simulink model "scheme_batch_op_regulation"  (R2025a)
settings: Solver=ode3  StartTime=0.0  StopTime=40  FixedStep=dt  RelTol=1e-3
values from neighbouring files (symbols this model uses):
  dt = 0.0001    [Planning_w_Adaptive.m]    (also in runBatchTests.m = 0.0005; tune_mrac_params.m = 0.01)
  map_scale = 0.5    [Planning_w_Adaptive.m]    (also in tune_mrac_params.m)
  N = -1 / (C_output_phi * inv(Am) * B)    [Planning_w_Adaptive.m]    (also in tune_mrac_params.m)
  op_space_pose_trajectory = zeros(4, 4, num_points)    [runBatchTests.m]
  waypoints = pathObj.States(:, 1:2)    [Planning_w_Adaptive.m]    (also in tune_mrac_params.m)
  x0 = zeros(10, 1)    [LQR_Control_generated.m]    (also in PID_LQR_PI_Loop.m = zeros(14, 1); Planning_w_Adaptive.m)
undefined symbols (not defined in the file or in its folder): control_params, initial_positions_rad, manipulator_time_vector, p, X, Y, Z
libraries: sm_lib x179, nesl_utility x28, fl_lib x3
(part 4 of 5)

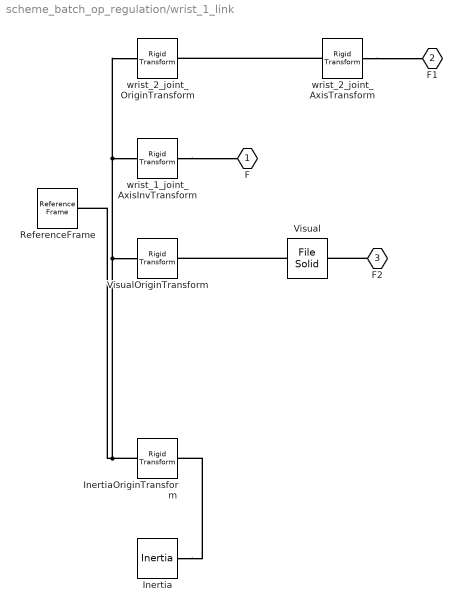
== system scheme_batch_op_regulation/wrist_1_link ==
  Inertia : sm_lib/Body Elements/Inertia  InertiaType=Custom  Mass=1.37  MassUnits=kg  CenterOfMass=[0, 0, 0]  CenterOfMassUnits=m  MomentsOfInertia=[0.00165491, 0.00126279, 0.00135962]  MomentsOfInertiaUnits=kg*m^2  ProductsOfInertia=[-0.00010157, -2.819999999999998e-06, 4.380000000000001e-06]  ProductsOfInertiaUnits=kg*m^2  GraphicType=None  MarkerShape=Inertia  MarkerSize=20  GraphicVisPropType=SimpleVisualProperties  GraphicDiffuseColor=[0.5 0.5 0.5]  GraphicOpacity=1  GraphicSpecularColor=[0.5 0.5 0.5 1.0]  GraphicAmbientColor=[0.15 0.15 0.15 1.0]  GraphicEmissiveColor=[0.0 0.0 0.0 1.0]  GraphicShininess=75
  InertiaOriginTransform : sm_lib/Frames and Transforms/Rigid Transform  RotationMethod=RotationSequence  FollAlignAxisA=+X  BaseAlignAxisA=+Y  FollAlignAxisB=+Y  BaseAlignAxisB=+Z  RotationStandardAxis=+Z  RotationAngle=0  RotationAngleUnits=deg  RotationArbitraryAxis=[0 0 1]  RotationSequenceAxes=BaseAxes  RotationSequence=XYZ  RotationSequenceAngles=[0, 0, 0]  RotationSequenceAnglesUnits=rad  RotationMatrix=[1 0 0;0 1 0;0 0 1]  Quaternion=[1 0 0 0]  TranslationMethod=Cartesian  TranslationCartesianOffset=[0, -0.01634, -0.0018]  TranslationCartesianOffsetUnits=m  TranslationStandardAxis=+Z  TranslationStandardOffset=0  TranslationStandardOffsetUnits=m  TranslationROffset=0  TranslationROffsetUnits=m  TranslationThetaOffset=0  TranslationThetaOffsetUnits=deg  TranslationZOffset=0  TranslationZOffsetUnits=m
  ReferenceFrame : sm_lib/Frames and Transforms/Reference Frame
  Visual : sm_lib/Body Elements/File Solid  ExtGeomFileName=C:\Users\robyr\Desktop\MatDrive\Published\FieldProject\generated\ros_packages\ur_description\meshes\ur5e\visual\wrist1.dae  UnitType=Custom  ExtGeomFileUnits=m  StepReaderType=HEX  ExportConvexHullGeometry=on  InertiaType=Custom  BasedOnType=DensityFromFile  Density=1000  DensityUnits=kg/m^3  Mass=0  MassUnits=kg  CenterOfMass=[0, 0, 0]  CenterOfMassUnits=m  MomentsOfInertia=[0, 0, 0]  MomentsOfInertiaUnits=kg*m^2  ProductsOfInertia=[0, 0, 0]  ProductsOfInertiaUnits=kg*m^2  GraphicType=FromGeometry  MarkerShape=Sphere  MarkerSize=10  GraphicVisPropType=SimpleVisualProperties  GraphicDiffuseColor=[0.5, 0.5, 0.5]  GraphicOpacity=1  GraphicSpecularColor=[0.5 0.5 0.5 1.0]  GraphicAmbientColor=[0.15 0.15 0.15 1.0]  GraphicEmissiveColor=[0.0 0.0 0.0 1.0]  GraphicShininess=75  DoExposeReferenceFrame=on  SerializedFrames=<Frames/>
  VisualOriginTransform : sm_lib/Frames and Transforms/Rigid Transform  RotationMethod=RotationSequence  FollAlignAxisA=+X  BaseAlignAxisA=+Y  FollAlignAxisB=+Y  BaseAlignAxisB=+Z  RotationStandardAxis=+Z  RotationAngle=0  RotationAngleUnits=deg  RotationArbitraryAxis=[0 0 1]  RotationSequenceAxes=BaseAxes  RotationSequence=XYZ  RotationSequenceAngles=[1.570796326794897, 0, 0]  RotationSequenceAnglesUnits=rad  RotationMatrix=[1 0 0;0 1 0;0 0 1]  Quaternion=[1 0 0 0]  TranslationMethod=Cartesian  TranslationCartesianOffset=[0, 0, -0.127]  TranslationCartesianOffsetUnits=m  TranslationStandardAxis=+Z  TranslationStandardOffset=0  TranslationStandardOffsetUnits=m  TranslationROffset=0  TranslationROffsetUnits=m  TranslationThetaOffset=0  TranslationThetaOffsetUnits=deg  TranslationZOffset=0  TranslationZOffsetUnits=m
  wrist_1_joint_AxisInvTransform : sm_lib/Frames and Transforms/Rigid Transform  RotationMethod=ArbitraryAxis  FollAlignAxisA=+X  BaseAlignAxisA=+Y  FollAlignAxisB=+Y  BaseAlignAxisB=+Z  RotationStandardAxis=+Z  RotationAngle=0  RotationAngleUnits=rad  RotationArbitraryAxis=[1, 0, 0]  RotationSequenceAxes=FollowerAxes  RotationSequence=XYX  RotationSequenceAngles=[0 0 0]  RotationSequenceAnglesUnits=deg  RotationMatrix=[1 0 0;0 1 0;0 0 1]  Quaternion=[1 0 0 0]  TranslationMethod=Cartesian  TranslationCartesianOffset=[0, 0, 0]  TranslationCartesianOffsetUnits=m  TranslationStandardAxis=+Z  TranslationStandardOffset=0  TranslationStandardOffsetUnits=m  TranslationROffset=0  TranslationROffsetUnits=m  TranslationThetaOffset=0  TranslationThetaOffsetUnits=deg  TranslationZOffset=0  TranslationZOffsetUnits=m
  wrist_2_joint_AxisTransform : sm_lib/Frames and Transforms/Rigid Transform  RotationMethod=ArbitraryAxis  FollAlignAxisA=+X  BaseAlignAxisA=+Y  FollAlignAxisB=+Y  BaseAlignAxisB=+Z  RotationStandardAxis=+Z  RotationAngle=0  RotationAngleUnits=rad  RotationArbitraryAxis=[1, 0, 0]  RotationSequenceAxes=FollowerAxes  RotationSequence=XYX  RotationSequenceAngles=[0 0 0]  RotationSequenceAnglesUnits=deg  RotationMatrix=[1 0 0;0 1 0;0 0 1]  Quaternion=[1 0 0 0]  TranslationMethod=Cartesian  TranslationCartesianOffset=[0, 0, 0]  TranslationCartesianOffsetUnits=m  TranslationStandardAxis=+Z  TranslationStandardOffset=0  TranslationStandardOffsetUnits=m  TranslationROffset=0  TranslationROffsetUnits=m  TranslationThetaOffset=0  TranslationThetaOffsetUnits=deg  TranslationZOffset=0  TranslationZOffsetUnits=m
  wrist_2_joint_OriginTransform : sm_lib/Frames and Transforms/Rigid Transform  RotationMethod=RotationSequence  FollAlignAxisA=+X  BaseAlignAxisA=+Y  FollAlignAxisB=+Y  BaseAlignAxisB=+Z  RotationStandardAxis=+Z  RotationAngle=0  RotationAngleUnits=deg  RotationArbitraryAxis=[0 0 1]  RotationSequenceAxes=BaseAxes  RotationSequence=XYZ  RotationSequenceAngles=[1.570796327, -0, 0]  RotationSequenceAnglesUnits=rad  RotationMatrix=[1 0 0;0 1 0;0 0 1]  Quaternion=[1 0 0 0]  TranslationMethod=Cartesian  TranslationCartesianOffset=[0, -0.0997, -2.044881182297852e-11]  TranslationCartesianOffsetUnits=m  TranslationStandardAxis=+Z  TranslationStandardOffset=0  TranslationStandardOffsetUnits=m  TranslationROffset=0  TranslationROffsetUnits=m  TranslationThetaOffset=0  TranslationThetaOffsetUnits=deg  TranslationZOffset=0  TranslationZOffsetUnits=m
  F : PMIOPort  Side=Left
  F1 : PMIOPort  Port=2  Side=Right
  F2 : PMIOPort  Port=3  Side=Left
  connections:
  Inertia/RConn1 -- InertiaOriginTransform/RConn1
  ReferenceFrame/RConn1 -- InertiaOriginTransform/LConn1 -- wrist_1_joint_AxisInvTransform/LConn1 -- wrist_2_joint_OriginTransform/LConn1 -- VisualOriginTransform/LConn1
  Visual/RConn1 -- VisualOriginTransform/RConn1
  wrist_1_joint_AxisInvTransform/RConn1 -- F/RConn1
  wrist_2_joint_AxisTransform/RConn1 -- F1/RConn1
  wrist_2_joint_AxisTransform/LConn1 -- wrist_2_joint_OriginTransform/RConn1
  F2/RConn1 -- Visual/LConn1

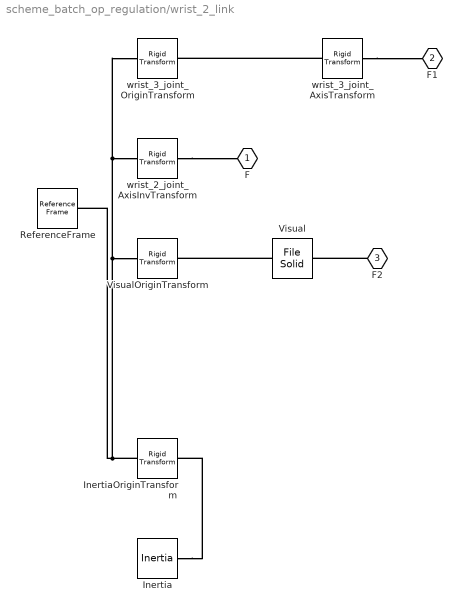
== system scheme_batch_op_regulation/wrist_2_link ==
  Inertia : sm_lib/Body Elements/Inertia  InertiaType=Custom  Mass=1.3  MassUnits=kg  CenterOfMass=[0, 0, 0]  CenterOfMassUnits=m  MomentsOfInertia=[0.00135617, 0.00096614, 0.00127827]  MomentsOfInertiaUnits=kg*m^2  ProductsOfInertia=[5.048000000000011e-05, 2.739999999999998e-06, 4.440000000000001e-06]  ProductsOfInertiaUnits=kg*m^2  GraphicType=None  MarkerShape=Inertia  MarkerSize=20  GraphicVisPropType=SimpleVisualProperties  GraphicDiffuseColor=[0.5 0.5 0.5]  GraphicOpacity=1  GraphicSpecularColor=[0.5 0.5 0.5 1.0]  GraphicAmbientColor=[0.15 0.15 0.15 1.0]  GraphicEmissiveColor=[0.0 0.0 0.0 1.0]  GraphicShininess=75
  InertiaOriginTransform : sm_lib/Frames and Transforms/Rigid Transform  RotationMethod=RotationSequence  FollAlignAxisA=+X  BaseAlignAxisA=+Y  FollAlignAxisB=+Y  BaseAlignAxisB=+Z  RotationStandardAxis=+Z  RotationAngle=0  RotationAngleUnits=deg  RotationArbitraryAxis=[0 0 1]  RotationSequenceAxes=BaseAxes  RotationSequence=XYZ  RotationSequenceAngles=[0, 0, 0]  RotationSequenceAnglesUnits=rad  RotationMatrix=[1 0 0;0 1 0;0 0 1]  Quaternion=[1 0 0 0]  TranslationMethod=Cartesian  TranslationCartesianOffset=[0, 0.01634, -0.0018]  TranslationCartesianOffsetUnits=m  TranslationStandardAxis=+Z  TranslationStandardOffset=0  TranslationStandardOffsetUnits=m  TranslationROffset=0  TranslationROffsetUnits=m  TranslationThetaOffset=0  TranslationThetaOffsetUnits=deg  TranslationZOffset=0  TranslationZOffsetUnits=m
  ReferenceFrame : sm_lib/Frames and Transforms/Reference Frame
  Visual : sm_lib/Body Elements/File Solid  ExtGeomFileName=C:\Users\robyr\Desktop\MatDrive\Published\FieldProject\generated\ros_packages\ur_description\meshes\ur5e\visual\wrist2.dae  UnitType=Custom  ExtGeomFileUnits=m  StepReaderType=HEX  ExportConvexHullGeometry=on  InertiaType=Custom  BasedOnType=DensityFromFile  Density=1000  DensityUnits=kg/m^3  Mass=0  MassUnits=kg  CenterOfMass=[0, 0, 0]  CenterOfMassUnits=m  MomentsOfInertia=[0, 0, 0]  MomentsOfInertiaUnits=kg*m^2  ProductsOfInertia=[0, 0, 0]  ProductsOfInertiaUnits=kg*m^2  GraphicType=FromGeometry  MarkerShape=Sphere  MarkerSize=10  GraphicVisPropType=SimpleVisualProperties  GraphicDiffuseColor=[0.5, 0.5, 0.5]  GraphicOpacity=1  GraphicSpecularColor=[0.5 0.5 0.5 1.0]  GraphicAmbientColor=[0.15 0.15 0.15 1.0]  GraphicEmissiveColor=[0.0 0.0 0.0 1.0]  GraphicShininess=75  DoExposeReferenceFrame=on  SerializedFrames=<Frames/>
  VisualOriginTransform : sm_lib/Frames and Transforms/Rigid Transform  RotationMethod=RotationSequence  FollAlignAxisA=+X  BaseAlignAxisA=+Y  FollAlignAxisB=+Y  BaseAlignAxisB=+Z  RotationStandardAxis=+Z  RotationAngle=0  RotationAngleUnits=deg  RotationArbitraryAxis=[0 0 1]  RotationSequenceAxes=BaseAxes  RotationSequence=XYZ  RotationSequenceAngles=[0, 0, 0]  RotationSequenceAnglesUnits=rad  RotationMatrix=[1 0 0;0 1 0;0 0 1]  Quaternion=[1 0 0 0]  TranslationMethod=Cartesian  TranslationCartesianOffset=[0, 0, -0.0997]  TranslationCartesianOffsetUnits=m  TranslationStandardAxis=+Z  TranslationStandardOffset=0  TranslationStandardOffsetUnits=m  TranslationROffset=0  TranslationROffsetUnits=m  TranslationThetaOffset=0  TranslationThetaOffsetUnits=deg  TranslationZOffset=0  TranslationZOffsetUnits=m
  wrist_2_joint_AxisInvTransform : sm_lib/Frames and Transforms/Rigid Transform  RotationMethod=ArbitraryAxis  FollAlignAxisA=+X  BaseAlignAxisA=+Y  FollAlignAxisB=+Y  BaseAlignAxisB=+Z  RotationStandardAxis=+Z  RotationAngle=0  RotationAngleUnits=rad  RotationArbitraryAxis=[1, 0, 0]  RotationSequenceAxes=FollowerAxes  RotationSequence=XYX  RotationSequenceAngles=[0 0 0]  RotationSequenceAnglesUnits=deg  RotationMatrix=[1 0 0;0 1 0;0 0 1]  Quaternion=[1 0 0 0]  TranslationMethod=Cartesian  TranslationCartesianOffset=[0, 0, 0]  TranslationCartesianOffsetUnits=m  TranslationStandardAxis=+Z  TranslationStandardOffset=0  TranslationStandardOffsetUnits=m  TranslationROffset=0  TranslationROffsetUnits=m  TranslationThetaOffset=0  TranslationThetaOffsetUnits=deg  TranslationZOffset=0  TranslationZOffsetUnits=m
  wrist_3_joint_AxisTransform : sm_lib/Frames and Transforms/Rigid Transform  RotationMethod=ArbitraryAxis  FollAlignAxisA=+X  BaseAlignAxisA=+Y  FollAlignAxisB=+Y  BaseAlignAxisB=+Z  RotationStandardAxis=+Z  RotationAngle=0  RotationAngleUnits=rad  RotationArbitraryAxis=[1, 0, 0]  RotationSequenceAxes=FollowerAxes  RotationSequence=XYX  RotationSequenceAngles=[0 0 0]  RotationSequenceAnglesUnits=deg  RotationMatrix=[1 0 0;0 1 0;0 0 1]  Quaternion=[1 0 0 0]  TranslationMethod=Cartesian  TranslationCartesianOffset=[0, 0, 0]  TranslationCartesianOffsetUnits=m  TranslationStandardAxis=+Z  TranslationStandardOffset=0  TranslationStandardOffsetUnits=m  TranslationROffset=0  TranslationROffsetUnits=m  TranslationThetaOffset=0  TranslationThetaOffsetUnits=deg  TranslationZOffset=0  TranslationZOffsetUnits=m
  wrist_3_joint_OriginTransform : sm_lib/Frames and Transforms/Rigid Transform  RotationMethod=RotationSequence  FollAlignAxisA=+X  BaseAlignAxisA=+Y  FollAlignAxisB=+Y  BaseAlignAxisB=+Z  RotationStandardAxis=+Z  RotationAngle=0  RotationAngleUnits=deg  RotationArbitraryAxis=[0 0 1]  RotationSequenceAxes=BaseAxes  RotationSequence=XYZ  RotationSequenceAngles=[-1.570796327, 1.224646799147353e-16, -1.224646799147353e-16]  RotationSequenceAnglesUnits=rad  RotationMatrix=[1 0 0;0 1 0;0 0 1]  Quaternion=[1 0 0 0]  TranslationMethod=Cartesian  TranslationCartesianOffset=[0, 0.09959999999999999, -2.042830148012698e-11]  TranslationCartesianOffsetUnits=m  TranslationStandardAxis=+Z  TranslationStandardOffset=0  TranslationStandardOffsetUnits=m  TranslationROffset=0  TranslationROffsetUnits=m  TranslationThetaOffset=0  TranslationThetaOffsetUnits=deg  TranslationZOffset=0  TranslationZOffsetUnits=m
  F : PMIOPort  Side=Left
  F1 : PMIOPort  Port=2  Side=Right
  F2 : PMIOPort  Port=3  Side=Left
  connections:
  Inertia/RConn1 -- InertiaOriginTransform/RConn1
  ReferenceFrame/RConn1 -- InertiaOriginTransform/LConn1 -- wrist_2_joint_AxisInvTransform/LConn1 -- wrist_3_joint_OriginTransform/LConn1 -- VisualOriginTransform/LConn1
  Visual/RConn1 -- VisualOriginTransform/RConn1
  wrist_2_joint_AxisInvTransform/RConn1 -- F/RConn1
  wrist_3_joint_AxisTransform/RConn1 -- F1/RConn1
  wrist_3_joint_AxisTransform/LConn1 -- wrist_3_joint_OriginTransform/RConn1
  F2/RConn1 -- Visual/LConn1

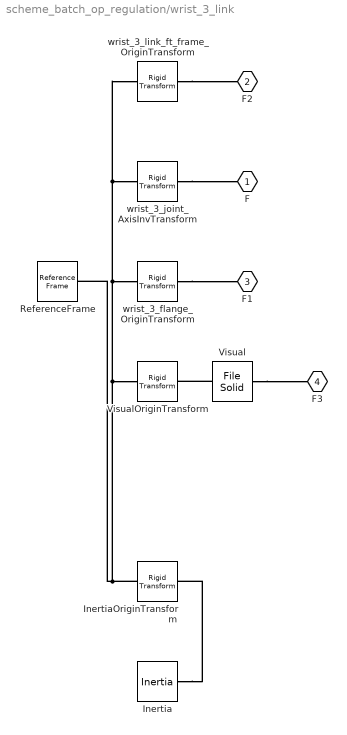
== system scheme_batch_op_regulation/wrist_3_link ==
  Inertia : sm_lib/Body Elements/Inertia  InertiaType=Custom  Mass=0.365  MassUnits=kg  CenterOfMass=[0, 0, 0]  CenterOfMassUnits=m  MomentsOfInertia=[0.00018694, 0.00018908, 0.00025756]  MomentsOfInertiaUnits=kg*m^2  ProductsOfInertia=[-9.2e-07, -1.7e-07, 5.999999999999999e-08]  ProductsOfInertiaUnits=kg*m^2  GraphicType=None  MarkerShape=Inertia  MarkerSize=20  GraphicVisPropType=SimpleVisualProperties  GraphicDiffuseColor=[0.5 0.5 0.5]  GraphicOpacity=1  GraphicSpecularColor=[0.5 0.5 0.5 1.0]  GraphicAmbientColor=[0.15 0.15 0.15 1.0]  GraphicEmissiveColor=[0.0 0.0 0.0 1.0]  GraphicShininess=75
  InertiaOriginTransform : sm_lib/Frames and Transforms/Rigid Transform  RotationMethod=RotationSequence  FollAlignAxisA=+X  BaseAlignAxisA=+Y  FollAlignAxisB=+Y  BaseAlignAxisB=+Z  RotationStandardAxis=+Z  RotationAngle=0  RotationAngleUnits=deg  RotationArbitraryAxis=[0 0 1]  RotationSequenceAxes=BaseAxes  RotationSequence=XYZ  RotationSequenceAngles=[0, 0, 0]  RotationSequenceAnglesUnits=rad  RotationMatrix=[1 0 0;0 1 0;0 0 1]  Quaternion=[1 0 0 0]  TranslationMethod=Cartesian  TranslationCartesianOffset=[0, 0, -0.001159]  TranslationCartesianOffsetUnits=m  TranslationStandardAxis=+Z  TranslationStandardOffset=0  TranslationStandardOffsetUnits=m  TranslationROffset=0  TranslationROffsetUnits=m  TranslationThetaOffset=0  TranslationThetaOffsetUnits=deg  TranslationZOffset=0  TranslationZOffsetUnits=m
  ReferenceFrame : sm_lib/Frames and Transforms/Reference Frame
  Visual : sm_lib/Body Elements/File Solid  ExtGeomFileName=C:\Users\robyr\Desktop\MatDrive\Published\FieldProject\generated\ros_packages\ur_description\meshes\ur5e\visual\wrist3.dae  UnitType=Custom  ExtGeomFileUnits=m  StepReaderType=HEX  ExportConvexHullGeometry=on  InertiaType=Custom  BasedOnType=DensityFromFile  Density=1000  DensityUnits=kg/m^3  Mass=0  MassUnits=kg  CenterOfMass=[0, 0, 0]  CenterOfMassUnits=m  MomentsOfInertia=[0, 0, 0]  MomentsOfInertiaUnits=kg*m^2  ProductsOfInertia=[0, 0, 0]  ProductsOfInertiaUnits=kg*m^2  GraphicType=FromGeometry  MarkerShape=Sphere  MarkerSize=10  GraphicVisPropType=SimpleVisualProperties  GraphicDiffuseColor=[0.5, 0.5, 0.5]  GraphicOpacity=1  GraphicSpecularColor=[0.5 0.5 0.5 1.0]  GraphicAmbientColor=[0.15 0.15 0.15 1.0]  GraphicEmissiveColor=[0.0 0.0 0.0 1.0]  GraphicShininess=75  DoExposeReferenceFrame=on  SerializedFrames=<Frames/>
  VisualOriginTransform : sm_lib/Frames and Transforms/Rigid Transform  RotationMethod=RotationSequence  FollAlignAxisA=+X  BaseAlignAxisA=+Y  FollAlignAxisB=+Y  BaseAlignAxisB=+Z  RotationStandardAxis=+Z  RotationAngle=0  RotationAngleUnits=deg  RotationArbitraryAxis=[0 0 1]  RotationSequenceAxes=BaseAxes  RotationSequence=XYZ  RotationSequenceAngles=[1.570796326794897, 0, 0]  RotationSequenceAnglesUnits=rad  RotationMatrix=[1 0 0;0 1 0;0 0 1]  Quaternion=[1 0 0 0]  TranslationMethod=Cartesian  TranslationCartesianOffset=[0, 0, -0.0989]  TranslationCartesianOffsetUnits=m  TranslationStandardAxis=+Z  TranslationStandardOffset=0  TranslationStandardOffsetUnits=m  TranslationROffset=0  TranslationROffsetUnits=m  TranslationThetaOffset=0  TranslationThetaOffsetUnits=deg  TranslationZOffset=0  TranslationZOffsetUnits=m
  wrist_3_flange_OriginTransform : sm_lib/Frames and Transforms/Rigid Transform  RotationMethod=RotationSequence  FollAlignAxisA=+X  BaseAlignAxisA=+Y  FollAlignAxisB=+Y  BaseAlignAxisB=+Z  RotationStandardAxis=+Z  RotationAngle=0  RotationAngleUnits=deg  RotationArbitraryAxis=[0 0 1]  RotationSequenceAxes=BaseAxes  RotationSequence=XYZ  RotationSequenceAngles=[-1.570796326794897, -1.570796326794897, 0]  RotationSequenceAnglesUnits=rad  RotationMatrix=[1 0 0;0 1 0;0 0 1]  Quaternion=[1 0 0 0]  TranslationMethod=Cartesian  TranslationCartesianOffset=[0, 0, 0]  TranslationCartesianOffsetUnits=m  TranslationStandardAxis=+Z  TranslationStandardOffset=0  TranslationStandardOffsetUnits=m  TranslationROffset=0  TranslationROffsetUnits=m  TranslationThetaOffset=0  TranslationThetaOffsetUnits=deg  TranslationZOffset=0  TranslationZOffsetUnits=m
  wrist_3_joint_AxisInvTransform : sm_lib/Frames and Transforms/Rigid Transform  RotationMethod=ArbitraryAxis  FollAlignAxisA=+X  BaseAlignAxisA=+Y  FollAlignAxisB=+Y  BaseAlignAxisB=+Z  RotationStandardAxis=+Z  RotationAngle=0  RotationAngleUnits=rad  RotationArbitraryAxis=[1, 0, 0]  RotationSequenceAxes=FollowerAxes  RotationSequence=XYX  RotationSequenceAngles=[0 0 0]  RotationSequenceAnglesUnits=deg  RotationMatrix=[1 0 0;0 1 0;0 0 1]  Quaternion=[1 0 0 0]  TranslationMethod=Cartesian  TranslationCartesianOffset=[0, 0, 0]  TranslationCartesianOffsetUnits=m  TranslationStandardAxis=+Z  TranslationStandardOffset=0  TranslationStandardOffsetUnits=m  TranslationROffset=0  TranslationROffsetUnits=m  TranslationThetaOffset=0  TranslationThetaOffsetUnits=deg  TranslationZOffset=0  TranslationZOffsetUnits=m
  wrist_3_link_ft_frame_OriginTransform : sm_lib/Frames and Transforms/Rigid Transform  RotationMethod=RotationSequence  FollAlignAxisA=+X  BaseAlignAxisA=+Y  FollAlignAxisB=+Y  BaseAlignAxisB=+Z  RotationStandardAxis=+Z  RotationAngle=0  RotationAngleUnits=deg  RotationArbitraryAxis=[0 0 1]  RotationSequenceAxes=BaseAxes  RotationSequence=XYZ  RotationSequenceAngles=[3.141592653589793, -0, 0]  RotationSequenceAnglesUnits=rad  RotationMatrix=[1 0 0;0 1 0;0 0 1]  Quaternion=[1 0 0 0]  TranslationMethod=Cartesian  TranslationCartesianOffset=[0, 0, 0]  TranslationCartesianOffsetUnits=m  TranslationStandardAxis=+Z  TranslationStandardOffset=0  TranslationStandardOffsetUnits=m  TranslationROffset=0  TranslationROffsetUnits=m  TranslationThetaOffset=0  TranslationThetaOffsetUnits=deg  TranslationZOffset=0  TranslationZOffsetUnits=m
  F : PMIOPort  Side=Left
  F2 : PMIOPort  Port=2  Side=Right
  F1 : PMIOPort  Port=3  Side=Right
  F3 : PMIOPort  Port=4  Side=Left
  connections:
  Inertia/RConn1 -- InertiaOriginTransform/RConn1
  ReferenceFrame/RConn1 -- InertiaOriginTransform/LConn1 -- wrist_3_joint_AxisInvTransform/LConn1 -- wrist_3_link_ft_frame_OriginTransform/LConn1 -- wrist_3_flange_OriginTransform/LConn1 -- VisualOriginTransform/LConn1
  Visual/RConn1 -- VisualOriginTransform/RConn1
  wrist_3_flange_OriginTransform/RConn1 -- F1/RConn1
  wrist_3_joint_AxisInvTransform/RConn1 -- F/RConn1
  wrist_3_link_ft_frame_OriginTransform/RConn1 -- F2/RConn1
  Visual/LConn1 -- F3/RConn1

== matlab function scheme_batch_op_regulation/MATLAB Function ==
  data: q_ref_gripper output; simscape_trajectory input; q_ref_manip output; q_op_integrated input; control_params parameter
function [q_ref_gripper,q_ref_manip ] = combine_joint_references(simscape_trajectory, q_op_integrated, control_params)
%
% This function combines a base joint-space position trajectory
% with an INTEGRATED operational-space correction command.
% It also separates the gripper command.
%
% INPUTS:
%   simscape_trajectory: (1x7) vector of joint POSITIONS from Simscape.
%   q_op_integrated:     (6x1) vector of joint POSITIONS from integrating
%                        the q_dot_command.
%
% OUTPUTS:
%   q_ref_manip:   (6x1) The final 6-joint position command.
%   q_ref_gripper: (1x1) The gripper command.
%

% --- 1. Ensure q_op_integrated is a 6x1 column vector ---
% (This helps prevent dimension mismatch errors)
q_op_integrated_col = reshape(q_op_integrated, 6, 1);

% --- 2. Extract the gripper command ---
% The 4th component of the simscape trajectory
q_ref_gripper = simscape_trajectory(4);

% --- 3. Extract the 6 manipulator joint references ---
% We take components 1, 2, 3, 5, 6, 7 and form a 6x1 column vector
q_ref_base_manip = [simscape_trajectory(1);
                    simscape_trajectory(2);
                    simscape_trajectory(3);
                    simscape_trajectory(5);
                    simscape_trajectory(6);
                    simscape_trajectory(7)];

% --- 4. Sum the base reference and the integrated correction ---
% This is the final position command for the 6 manipulator joints
q_ref_manip = q_ref_base_manip + control_params.k_op*q_op_integrated_col;

end

== matlab function scheme_batch_op_regulation/Smart LookUpTable ==
  settings: updateMethod=DISCRETE
  data: T_desired output; EUL output; t_in input; op_space_pose_trajectory parameter; manipulator_time_vector parameter; P output
function [T_desired, EUL, P] = get_pose_from_trajectory(t_in, op_space_pose_trajectory, manipulator_time_vector)
% =========================================================================
% TRAJECTORY INTERPOLATOR AND POSE SPLITTER (v4.1 - Column Vector Fix)
%
% This version transposes the EUL output to be a column vector [3x1]
% to match the expectation of downstream Simulink blocks like Demux.
% =========================================================================
    % For Coder compatibility, explicitly define the output sizes.
    P = zeros(3, 1);
    % FIX 1: Initialize EUL as a 3x1 column vector.
    EUL = zeros(3, 1);
    T_desired = eye(4);
    % Use a persistent variable to show warnings only once per simulation.
    persistent has_warned;
    if isempty(has_warned)
        has_warned = false;
    end

    % --- 1. Input Sanity Checks ---
    if isnan(t_in)
        if ~has_warned
            warning('Input time t_in is NaN. Outputting a zero pose.');
            has_warned = true;
        end
        return; % Exit with P and EUL as zeros
    end
    
    if isempty(manipulator_time_vector) || isempty(op_space_pose_trajectory)
        if ~has_warned
            warning('Trajectory data is empty. Outputting a zero pose.');
            has_warned = true;
        end
        return; % Exit with P and EUL as zeros
    end

    % --- 2. Data Formatting ---
    if isrow(manipulator_time_vector)
        manipulator_time_vector = manipulator_time_vector';
    end

    % --- 3. Interpolation ---
    if isscalar(manipulator_time_vector)
        T_interpolated = op_space_pose_trajectory(:,:,1);
    else
        num_points = size(op_space_pose_trajectory, 3);
        data_reshaped = reshape(op_space_pose_trajectory, 16, num_points)';
        
        interpolated_row = interp1(manipulator_time_vector, data_reshaped, t_in, 'linear', 'extrap');
        
        if any(isnan(interpolated_row))
             if ~has_warned
                warning('Interpolation resulted in NaN. Holding first pose as fallback.');
                has_warned = true;
             end
             T_interpolated = op_space_pose_trajectory(:,:,1);
        else
             T_interpolated = reshape(interpolated_row, 4, 4);
        end
    end
    
    % --- 4. Split the Result into Position and Euler Angles ---
    P = T_interpolated(1:3, 4);
    R = T_interpolated(1:3, 1:3);
    T_desired = T_interpolated;
    
    % FIX 2: Transpose the output of rotm2eul to create a column vector.
    EUL = rotm2eul(R, 'ZYX')'; % <-- The fix is the transpose operator '

end

== matlab function scheme_batch_op_regulation/OP SPACE CONTROLLER/MATLAB Function3 ==
  data: T_desired input; x_ballbot input; q_manip_actual input; q_dot_command output; error_pos output
function [q_dot_command,error_pos] = operational_space_controller(T_desired, x_ballbot, q_manip_actual)
% =========================================================================
% OPERATIONAL SPACE CONTROLLER (v5.1 - Final Coder-Safe Wrapper)
%
% This version correctly initializes the output variable before calling the
% extrinsic function, which is required for code generation.
% =========================================================================

    % --- Coder Directives ---
    coder.extrinsic('loadAndConfigureRobot', 'compute_op_space_velocities', 'disp');

    % --- Define persistent variables ---
    persistent robotModel p;

    % --- Initialization Block (runs only ONCE) ---
    if isempty(robotModel)
        disp('Controller Wrapper: Loading robot model and parameters...');
        robotModel = loadAndConfigureRobot('UR5e.urdf');
        p.h_U = 0.50;
        p.r_S = 0.1145;
        disp('Controller Wrapper initialized.');
    end

    % --- Main Control Call ---
    
    % FIX: Initialize the output variable with a known type and size (6x1 double).
    % This tells the Coder what to expect from the extrinsic function call.
    q_dot_command = zeros(6, 1);
    error_pos     = zeros(3, 1);
    
    % Call the single extrinsic "black box" function to do all the calculations.
    %error_pos = compute_error(robotModel, p, T_desired, x_ballbot, q_manip_actual);
    [q_dot_command,error_pos] = compute_op_space_velocities(robotModel, p, T_desired, x_ballbot, q_manip_actual);


end

== matlab function scheme_batch_op_regulation/EQ generator ==
  settings: updateMethod=DISCRETE
  data: phi_dot_c input; external_wrench input; theta_EQ output; p parameter; tau_EQ output
function [theta_EQ, tau_EQ] = compute_equilibrium_fsolve_2D(phi_dot_c, external_wrench, p)
% =========================================================================
% COMPUTE_EQUILIBRIUM_FSOLVE (v8 - Refactored)
%
% This function is now a pure solver. It calculates the equilibrium tilt
% angles (theta_EQ) and torques (tau_EQ) required to achieve a given
% wheel speed command (phi_dot_c) while under the influence of an
% external wrench.
%
% INPUTS:
%   x                - Current 10x1 state vector of the system.
%   phi_dot_c        - 2x1 desired wheel speed command [phi_dot_c_y; phi_dot_c_x].
%   external_wrench  - External forces and torques.
%   p                - Struct with system parameters.
% =========================================================================

% Use persistent variables for "warm-starting" the solver.
persistent prev_solution_x prev_solution_y;
if isempty(prev_solution_x)
    prev_solution_x = [0; 0]; % [theta_x; tau_x]
    prev_solution_y = [0; 0]; % [theta_y; tau_y]
end

%% === SECTION 1: UNPACK SPEED COMMAND ===
% The velocity command is now an input to the function.
phi_dot_c_y = phi_dot_c(1);
phi_dot_c_x = phi_dot_c(2);

%% === SECTION 2: FSOLVE FOR EQUILIBRIUM (CODER-FRIENDLY) ===
options = optimoptions('fsolve', 'Display', 'off', ...
                       'Algorithm', 'levenberg-marquardt', ...
                       'FunctionTolerance', 1e-6, ...
                       'StepTolerance', 1e-6, ...
                       'MaxIterations', 25);

% --- Solve for Pitch (Y-Z) Plane ---
up_y = [external_wrench(1); external_wrench(3); external_wrench(5)]; % [Fpx; Fpz; tau_py]
[current_solution_y, ~, exitflag_y] = fsolve(@(x_solve) equilibrium_residual_Y(x_solve, up_y, phi_dot_c_y, p), prev_solution_y, options);
if exitflag_y <= 0
    current_solution_y = prev_solution_y; % Fallback to previous solution on failure
end
theta_EQy_calc = current_solution_y(1);
tau_EQy_calc = current_solution_y(2);
prev_solution_y = current_solution_y;

% --- Solve for Roll (X-Z) Plane ---
up_x = [external_wrench(2); external_wrench(3); external_wrench(4)]; % [Fpy; Fpz; tau_px]
[current_solution_x, ~, exitflag_x] = fsolve(@(x_solve) equilibrium_residual_X(x_solve, up_x, phi_dot_c_x, p), prev_solution_x, options);
if exitflag_x <= 0
    current_solution_x = prev_solution_x; % Fallback
end
theta_EQx_calc = current_solution_x(1);
tau_EQx_calc = current_solution_x(2);
prev_solution_x = current_solution_x;

%% === SECTION 3: ASSEMBLE OUTPUTS ===
theta_EQ = [theta_EQx_calc; theta_EQy_calc];
tau_EQ = [tau_EQx_calc; tau_EQy_calc];

end

% --- Nested functions for solver residuals (unchanged) ---
function r = equilibrium_residual_Y(x_solve, upy, phi_dot_c, p)
    theta_eq = x_solve(1); tau_eq = x_solve(2);
    state_vec = [0; theta_eq; 0; 0; 0; 0; 0; 0; 0; phi_dot_c];
    tau_vec = [0; tau_eq; 0];
    wrench_vec = [upy(1); 0; upy(2); 0; upy(3)];
    dx = stateDerivative3D_with_exforce(state_vec, p, tau_vec, wrench_vec);
    r = [dx(7); dx(10)];
end

function r = equilibrium_residual_X(x_solve, upx, phi_dot_c, p)
    theta_eq = x_solve(1); tau_eq = x_solve(2);
    state_vec = [theta_eq; 0; 0; 0; 0; 0; 0; 0; phi_dot_c; 0];
    tau_vec = [tau_eq; 0; 0];
    wrench_vec = [0; upx(1); upx(2); upx(3); 0];
    dx = stateDerivative3D_with_exforce(state_vec, p, tau_vec, wrench_vec);
    r = [dx(6); dx(9)];
end

function dx = stateDerivative3D_with_exforce(x, p, tau, wrench_ext)
    % MODIFICATION 1: The function now accepts a 4th argument, 'wrench_ext',
    % which is a vector containing the external forces and torques from Simulink.
    
    % Unpack state vector (10 elements)
    theta_x = x(1); dot_theta_x = x(6);
    theta_y = x(2); dot_theta_y = x(7);
    theta_z = x(3); dot_theta_z = x(8);
    % phi_x   = x(4); % Not needed for dynamics
    % phi_y   = x(5); % Not needed for dynamics
    dot_phi_x   = x(9);
    dot_phi_y   = x(10);
    
    % Unpack input torques
    tau_x = tau(1);
    tau_y = tau(2);
    tau_z = tau(3);

     % Unpack the external wrench vector from the new input ---
    % Expected order: [F_px, F_py, F_pz, tau_px, tau_py]
    F_px   = wrench_ext(1);
    F_py   = wrench_ext(2);
    F_pz   = wrench_ext(3);
    tau_px = wrench_ext(4);
    tau_py = wrench_ext(5);

    % --- Prepare arguments for auto-generated functions ---
    % Create separate parameter vectors for each plane, now including h_app
    % Note: I_Ux is for roll, I_Uy is for pitch.
    params_arg_roll = [p.m_U,  p.I_Uy, p.I_Ux, p.l_U, p.m_S, p.I_S, p.r_S, p.g, p.h_app, p.b_theta, p.b_phi];
    params_arg_pitch = [p.m_U, p.I_Uy, p.I_Ux, p.l_U, p.m_S, p.I_S, p.r_S, p.g,p.h_app, p.b_theta, p.b_phi];
    
    external_vars_x = [F_py, F_pz, tau_px]; % For Roll dynamics
    external_vars_y = [F_px, F_pz, tau_py]; % For Pitch dynamics

    % --- X-Z Plane (Roll) Dynamics ---
    states_arg_x = [theta_x, dot_theta_x, dot_phi_x];
    inputs_arg_x = [tau_x];
    ddot_theta_x = copy_autogen_ddot_theta_x(states_arg_x, inputs_arg_x, params_arg_roll, external_vars_x);
    ddot_phi_x   = copy_autogen_ddot_phi_x(states_arg_x, inputs_arg_x, params_arg_roll, external_vars_x);
    

    % --- Y-Z Plane (Pitch) Dynamics ---
    states_arg_y = [theta_y, dot_theta_y, dot_phi_y];
    inputs_arg_y = [tau_y];
    ddot_theta_y = copy_autogen_ddot_theta_y(states_arg_y, inputs_arg_y, params_arg_pitch, external_vars_y);
    ddot_phi_y   = copy_autogen_ddot_phi_y(states_arg_y, inputs_arg_y, params_arg_pitch, external_vars_y);
    
    % --- Transversal Plane Dynamics (Yaw) ---
    % external forces at the center of the top surface are assumed not to produce yaw torque.
    ddot_theta_z = (tau_z - p.fz * dot_theta_z) / p.Iz;
    
    % --- Assemble the state derivative vector dx ---
    dx = [
        dot_theta_x;    % dx(1) = d(theta_x)/dt
        dot_theta_y;    % dx(2) = d(theta_y)/dt
        dot_theta_z;    % dx(3) = d(theta_z)/dt
        dot_phi_x;      % dx(4) = d(phi_x)/dt
        dot_phi_y;      % dx(5) = d(phi_y)/dt
        ddot_theta_x;   % dx(6) = d(dot_theta_x)/dt
        ddot_theta_y;   % dx(7) = d(dot_theta_y)/dt
        ddot_theta_z;   % dx(8) = d(dot_theta_z)/dt
        ddot_phi_x;     % dx(9) = d(dot_phi_x)/dt
        ddot_phi_y;     % dx(10)= d(dot_phi_y)/dt
    ];
end

== matlab function scheme_batch_op_regulation/LQR iHACS  ==
  settings: updateMethod=DISCRETE
  data: x input; tau output; dot_phi_cmd input; p parameter; control_params parameter; dt parameter; tau_ey output; tau_r output; tau_ex output; theta_EQ input; tau_ff_new output; tau_EQ input; sim_time input
function [tau, tau_ey, tau_r, tau_ex, tau_ff_new] = calculate_motor_torques(x, dot_phi_cmd, p, control_params, dt, theta_EQ, tau_EQ, sim_time)
% =========================================================================
% Ballbot Motor Torque Calculator (Inner Loop Controller)
%
% This function takes a desired wheel speed command and calculates the
% final motor torques using a cascaded LQR and PI control structure,
% compensated with feedforward equilibrium values.
%
% INPUTS:
%   x              (10x1): State vector
%   dot_phi_cmd    (2x1):  Desired wheel speed command [dot_phi_cmd_y; dot_phi_cmd_x]
%   p              (struct): System physical parameters
%   control_params (struct): Controller gains (K, Kp_inner, Ki_inner)
%   dt             (double): Controller sample time
%   theta_EQ       (2x1): Equilibrium tilt angles [theta_EQ_x; theta_EQ_y]
%   tau_EQ         (2x1): Equilibrium feedforward torques [tau_EQ_x; tau_EQ_y]
%   sim_time       (double): Current simulation time
% =========================================================================
persistent dot_phi_ref_old;
persistent integral_speed_error_old;
if isempty(dot_phi_ref_old)
    dot_phi_ref_old = zeros(2,1);
    integral_speed_error_old = zeros(2,1);
end

% --- UNPACK PARAMETERS, STATES, and INPUTS ---
K = control_params.K;
Kp_inner = control_params.Kp_inner;
Ki_inner = control_params.Ki_inner;
theta_x = x(1); dot_theta_x = x(6);
theta_y = x(2); dot_theta_y = x(7);
phi_x   = x(4); dot_phi_x   = x(9);
phi_y   = x(5); dot_phi_y   = x(10);
theta_EQ_x = theta_EQ(1);
theta_EQ_y = theta_EQ(2);
tau_EQ_x_raw   = tau_EQ(1);
tau_EQ_y_raw   = tau_EQ(2);

% Unpack the input speed command
dot_phi_cmd_y = dot_phi_cmd(1);
dot_phi_cmd_x = dot_phi_cmd(2);

%% --- FEEDBACK CONTROLLER (LQR + PI) ---
% --- LQR for stabilization ---
state_y = [theta_y; phi_y; dot_theta_y; dot_phi_y];
command_state_y = [theta_EQ_y; phi_y; 0; dot_phi_cmd_y];
tau_ry = -K * (state_y - command_state_y);

state_x = [theta_x; phi_x; dot_theta_x; dot_phi_x];
command_state_x = [theta_EQ_x; phi_x; 0; dot_phi_cmd_x];
tau_rx = -K * (state_x - command_state_x);
tau_z = 0;

% --- Inner PI loop speed controller ---
tau_r = [tau_rx; tau_ry; tau_z];
dx_ref = stateDerivative3D_with_exforce(x(1:10), p, tau_r, zeros(5,1));
ddot_phi_x_ref = dx_ref(9);
ddot_phi_y_ref = dx_ref(10);
dot_phi_x_ref = dot_phi_ref_old(1) + ddot_phi_x_ref * dt;
dot_phi_y_ref = dot_phi_ref_old(2) + ddot_phi_y_ref * dt;
speed_error_x = dot_phi_x_ref - dot_phi_x;
speed_error_y = dot_phi_y_ref - dot_phi_y;
int_err_vx = integral_speed_error_old(1);
int_err_vy = integral_speed_error_old(2);
tau_ex = Kp_inner * speed_error_x + Ki_inner * int_err_vx;
tau_ey = Kp_inner * speed_error_y + Ki_inner * int_err_vy;

%% --- FINAL TORQUE COMMAND ---
% Combine Feedback (LQR + PI) and Feedforward (Equilibrium Torque)
if sim_time < 0.1
    tau_EQ_x = 0;
    tau_EQ_y = 0;
else
    tau_EQ_x = tau_EQ_x_raw;
    tau_EQ_y = tau_EQ_y_raw;
end
tau_ff_new = [tau_EQ_x; tau_EQ_y; 0];
tau_x = tau_rx + tau_ex + tau_EQ_x;
tau_y = tau_ry + tau_ey + tau_EQ_y;
tau_z = 0;
tau = [tau_x; tau_y; tau_z];

% --- UPDATE PERSISTENT VARIABLES ---
integral_speed_error_old = integral_speed_error_old + [speed_error_x; speed_error_y] * dt;
dot_phi_ref_old = [dot_phi_x_ref; dot_phi_y_ref];

end

function dx = stateDerivative3D_with_exforce(x, p, tau, wrench_ext)
    % MODIFICATION 1: The function now accepts a 4th argument, 'wrench_ext',
    % which is a vector containing the external forces and torques from Simulink.
    
    % Unpack state vector (10 elements)
    theta_x = x(1); dot_theta_x = x(6);
    theta_y = x(2); dot_theta_y = x(7);
    theta_z = x(3); dot_theta_z = x(8);
    % phi_x   = x(4); % Not needed for dynamics
    % phi_y   = x(5); % Not needed for dynamics
    dot_phi_x   = x(9);
    dot_phi_y   = x(10);
    
    % Unpack input torques
    tau_x = tau(1);
    tau_y = tau(2);
    tau_z = tau(3);

     % Unpack the external wrench vector from the new input ---
    % Expected order: [F_px, F_py, F_pz, tau_px, tau_py]
    F_px   = wrench_ext(1);
    F_py   = wrench_ext(2);
    F_pz   = wrench_ext(3);
    tau_px = wrench_ext(4);
    tau_py = wrench_ext(5);

    % --- Prepare arguments for auto-generated functions ---
    % Create separate parameter vectors for each plane, now including h_app
    % Note: I_Ux is for roll, I_Uy is for pitch.
    params_arg_roll = [p.m_U,  p.I_Uy, p.I_Ux, p.l_U, p.m_S, p.I_S, p.r_S, p.g, p.h_app, p.b_theta, p.b_phi];
    params_arg_pitch = [p.m_U, p.I_Uy, p.I_Ux, p.l_U, p.m_S, p.I_S, p.r_S, p.g,p.h_app, p.b_theta, p.b_phi];
    
    external_vars_x = [F_py, F_pz, tau_px]; % For Roll dynamics
    external_vars_y = [F_px, F_pz, tau_py]; % For Pitch dynamics

    % --- X-Z Plane (Roll) Dynamics ---
    states_arg_x = [theta_x, dot_theta_x, dot_phi_x];
    inputs_arg_x = [tau_x];
    ddot_theta_x = copy_autogen_ddot_theta_x(states_arg_x, inputs_arg_x, params_arg_roll, external_vars_x);
    ddot_phi_x   = copy_autogen_ddot_phi_x(states_arg_x, inputs_arg_x, params_arg_roll, external_vars_x);
    

    % --- Y-Z Plane (Pitch) Dynamics ---
    states_arg_y = [theta_y, dot_theta_y, dot_phi_y];
    inputs_arg_y = [tau_y];
    ddot_theta_y = copy_autogen_ddot_theta_y(states_arg_y, inputs_arg_y, params_arg_pitch, external_vars_y);
    ddot_phi_y   = copy_autogen_ddot_phi_y(states_arg_y, inputs_arg_y, params_arg_pitch, external_vars_y);
    
    % --- Transversal Plane Dynamics (Yaw) ---
    % external forces at the center of the top surface are assumed not to produce yaw torque.
    ddot_theta_z = (tau_z - p.fz * dot_theta_z) / p.Iz;
    
    % --- Assemble the state derivative vector dx ---
    dx = [
        dot_theta_x;    % dx(1) = d(theta_x)/dt
        dot_theta_y;    % dx(2) = d(theta_y)/dt
        dot_theta_z;    % dx(3) = d(theta_z)/dt
        dot_phi_x;      % dx(4) = d(phi_x)/dt
        dot_phi_y;      % dx(5) = d(phi_y)/dt
        ddot_theta_x;   % dx(6) = d(dot_theta_x)/dt
        ddot_theta_y;   % dx(7) = d(dot_theta_y)/dt
        ddot_theta_z;   % dx(8) = d(dot_theta_z)/dt
        ddot_phi_x;     % dx(9) = d(dot_phi_x)/dt
        ddot_phi_y;     % dx(10)= d(dot_phi_y)/dt
    ];
end

== matlab function scheme_batch_op_regulation/LQR Controller1 ==
  settings: updateMethod=DISCRETE
  data: x input; tau output; waypoints input; p parameter; control_params parameter; map_scale parameter; dt parameter; tau_ey output; tau_r output; tau_ex output; external_wrench input; tau_ff output
function [tau, tau_ey, tau_r,tau_ex,tau_ff] = fcn(x, waypoints, p, control_params, map_scale, dt, external_wrench)
persistent current_waypoint_idx;
persistent dot_phi_ref_old; 
persistent integral_speed_error_old;

if isempty(current_waypoint_idx)
    current_waypoint_idx = 1;
    dot_phi_ref_old = zeros(2,1);
    integral_speed_error_old = zeros(2,1);
end

 % --- WAYPOINT NAVIGATION ---
waypoint_reach_threshold = 0.15 * map_scale;
p_target = waypoints(current_waypoint_idx, :)';
p_current = [p.r_S * x(5); -p.r_S * x(4)];
distance_to_target = norm(p_current - p_target);
if (distance_to_target < waypoint_reach_threshold) && (current_waypoint_idx < size(waypoints, 1))
    current_waypoint_idx = current_waypoint_idx + 1;
end

 % --- UNPACK PARAMETERS AND STATES  ---
K = control_params.K; Kp_pos = control_params.Kp_pos; Kp_inner = control_params.Kp_inner; Ki_inner = control_params.Ki_inner;
theta_x = x(1); dot_theta_x = x(6);
theta_y = x(2); dot_theta_y = x(7);
phi_x = x(4); dot_phi_x = x(9);
phi_y = x(5); dot_phi_y = x(10);

% --- FEEDBACK CONTROLLER (LQR + PI) ---
% Position controller
error_pos = p_target - p_current;
v_cmd = Kp_pos * error_pos;
dot_phi_cmd_y = v_cmd(1) / p.r_S;
dot_phi_cmd_x = -v_cmd(2) / p.r_S;

% LQR for stabilization
state_y = [theta_y; phi_y; dot_theta_y; dot_phi_y];
command_state_y = [0; phi_y; 0; dot_phi_cmd_y];
tau_ry = -K * (state_y - command_state_y);
state_x = [theta_x; phi_x; dot_theta_x; dot_phi_x];
command_state_x = [0; phi_x; 0; dot_phi_cmd_x];
tau_rx = -K * (state_x - command_state_x);
tau_z = 0;

 % Inner loop speed controller
tau_r = [tau_rx; tau_ry; tau_z];
dx_ref = stateDerivative3D_with_exforce(x(1:10), p, tau_r, zeros(5,1));
ddot_phi_x_ref = dx_ref(9);
ddot_phi_y_ref = dx_ref(10);

dot_phi_x_ref = dot_phi_ref_old(1) + ddot_phi_x_ref * dt;
dot_phi_y_ref = dot_phi_ref_old(2) + ddot_phi_y_ref * dt;

speed_error_x = dot_phi_x_ref - dot_phi_x;
speed_error_y = dot_phi_y_ref - dot_phi_y;
int_err_vx = integral_speed_error_old(1);
int_err_vy = integral_speed_error_old(2);
tau_ex = Kp_inner * speed_error_x + Ki_inner * int_err_vx;
tau_ey = Kp_inner * speed_error_y + Ki_inner * int_err_vy;

% --- NEW: FEEDFORWARD CONTROLLER FOR DISTURBANCE REJECTION ---
% 1. Assemble the generalized coordinate vector q_bot
q_bot = [theta_x; theta_y; phi_x; phi_y];

% 2. Call the feedforward controller to get cancellation torques
tau_ff = feedforwardController(q_bot, external_wrench, p);
% *****************************************************************

% --- FINAL TORQUE COMMAND (Combine Feedback and Feedforward) ---
tau_x = tau_rx + tau_ex + tau_ff(1); % Add feedforward torque for x-axis
tau_y = tau_ry + tau_ey + tau_ff(2); % Add feedforward torque for y-axis
tau_z = tau_ff(3);

tau = [tau_x; tau_y; tau_z];

% --- UPDATE PERSISTENT VARIABLES (No changes here) ---
integral_speed_error_old = integral_speed_error_old + [speed_error_x; speed_error_y] * dt;
dot_phi_ref_old = [dot_phi_x_ref; dot_phi_y_ref];

end

function dx = stateDerivative3D_with_exforce(x, p, tau, wrench_ext)
    theta_x = x(1); dot_theta_x = x(6);
    theta_y = x(2); dot_theta_y = x(7);
    theta_z = x(3); dot_theta_z = x(8);
    % phi_x   = x(4); % Not needed for dynamics
    % phi_y   = x(5); % Not needed for dynamics
    dot_phi_x   = x(9);
    dot_phi_y   = x(10);
    
    % Unpack input torques
    tau_x = tau(1);
    tau_y = tau(2);
    tau_z = tau(3);

     % Unpack the external wrench vector from the new input ---
    % Expected order: [F_px, F_py, F_pz, tau_px, tau_py]
    F_px   = wrench_ext(1);
    F_py   = wrench_ext(2);
    F_pz   = wrench_ext(3);
    tau_px = wrench_ext(4);
    tau_py = wrench_ext(5);

    % --- Prepare arguments for auto-generated functions ---
    % Create separate parameter vectors for each plane, now including h_app
    % Note: I_Ux is for roll, I_Uy is for pitch.
    params_arg_roll = [p.m_U,  p.I_Uy, p.I_Ux, p.l_U, p.m_S, p.I_S, p.r_S, p.g, p.h_app, p.b_theta, p.b_phi];
    params_arg_pitch = [p.m_U, p.I_Uy, p.I_Ux, p.l_U, p.m_S, p.I_S, p.r_S, p.g,p.h_app, p.b_theta, p.b_phi];
    
    external_vars_x = [F_py, F_pz, tau_px]; % For Roll dynamics
    external_vars_y = [F_px, F_pz, tau_py]; % For Pitch dynamics

    % --- X-Z Plane (Roll) Dynamics ---
    states_arg_x = [theta_x, dot_theta_x, dot_phi_x];
    inputs_arg_x = [tau_x];
    ddot_theta_x = copy_autogen_ddot_theta_x(states_arg_x, inputs_arg_x, params_arg_roll, external_vars_x);
    ddot_phi_x   = copy_autogen_ddot_phi_x(states_arg_x, inputs_arg_x, params_arg_roll, external_vars_x);
    

    % --- Y-Z Plane (Pitch) Dynamics ---
    states_arg_y = [theta_y, dot_theta_y, dot_phi_y];
    inputs_arg_y = [tau_y];
    ddot_theta_y = copy_autogen_ddot_theta_y(states_arg_y, inputs_arg_y, params_arg_pitch, external_vars_y);
    ddot_phi_y   = copy_autogen_ddot_phi_y(states_arg_y, inputs_arg_y, params_arg_pitch, external_vars_y);
    
    % --- Transversal Plane Dynamics (Yaw) ---
    % external forces at the center of the top surface are assumed not to produce yaw torque.
    ddot_theta_z = (tau_z - p.fz * dot_theta_z) / p.Iz;
    
    % --- Assemble the state derivative vector dx ---
    dx = [
        dot_theta_x;    % dx(1) = d(theta_x)/dt
        dot_theta_y;    % dx(2) = d(theta_y)/dt
        dot_theta_z;    % dx(3) = d(theta_z)/dt
        dot_phi_x;      % dx(4) = d(phi_x)/dt
        dot_phi_y;      % dx(5) = d(phi_y)/dt
        ddot_theta_x;   % dx(6) = d(dot_theta_x)/dt
        ddot_theta_y;   % dx(7) = d(dot_theta_y)/dt
        ddot_theta_z;   % dx(8) = d(dot_theta_z)/dt
        ddot_phi_x;     % dx(9) = d(dot_phi_x)/dt
        ddot_phi_y;     % dx(10)= d(dot_phi_y)/dt
    ];
end

function tau_ff = feedforwardController(q_bot, external_wrench, p)
    % feedforwardController
    % Calculates the feedforward torques to counteract an external wrench, including yaw torque.
    %
    % Inputs:
    %   q_bot:           Current generalized coordinates [theta_x; theta_y; phi_x; phi_y]
    %   external_wrench: Measured 6x1 wrench [Fx; Fy; Fz; Tx; Ty; Tz]
    %   p:               Struct of system parameters
    %
    % Output:
    %   tau_ff:          3x1 vector of feedforward torques [tau_ff_x; tau_ff_y; tau_ff_z]

    % Get geometric parameters
    R = p.r_S;
    h = p.h_app;

    % 1. Calculate the Jacobian for the roll/pitch dynamics
    % This part remains unchanged as J relates forces and roll/pitch torques
    % to the 4 generalized coordinates.
    J = calculateJacobian(q_bot, R, h);

    % 2. Calculate the generalized disturbance forces (d) for roll/pitch
    % We use the full 6x1 external wrench vector.
    d = J' * external_wrench;

    % 3. Map generalized forces to feedforward motor torques
    % d(1) is the disturbance torque on theta_x (roll)
    % d(2) is the disturbance torque on theta_y (pitch)
    tau_ff_x = d(1);
    tau_ff_y = d(2);
    
    % --- MODIFIED LOGIC FOR YAW ---
    % The external yaw torque (Tz) is the 6th element of the wrench vector.
    % external yaw torque Tz is already aligned with the yaw control axis tau_z
    %tau_ff_z = external_wrench(6);
    tau_ff_z = 0;
    
    tau_ff = [tau_ff_x; tau_ff_y; tau_ff_z];
end

== matlab function scheme_batch_op_regulation/BallBot Plant1/MATLAB Function ==
  data: dx output; x input; p parameter; tau input; wrench_ext input
function dx = stateDerivative3D_with_exforce(x, p, tau, wrench_ext)
    % MODIFICATION 1: The function now accepts a 4th argument, 'wrench_ext',
    % which is a vector containing the external forces and torques from Simulink.
    
    % Unpack state vector (10 elements)
    theta_x = x(1); dot_theta_x = x(6);
    theta_y = x(2); dot_theta_y = x(7);
    theta_z = x(3); dot_theta_z = x(8);
    % phi_x   = x(4); % Not needed for dynamics
    % phi_y   = x(5); % Not needed for dynamics
    dot_phi_x   = x(9);
    dot_phi_y   = x(10);
    
    % Unpack input torques
    tau_x = tau(1);
    tau_y = tau(2);
    tau_z = tau(3);

     % Unpack the external wrench vector from the new input ---
    % Expected order: [F_px, F_py, F_pz, tau_px, tau_py]
    F_px   = wrench_ext(1);
    F_py   = wrench_ext(2);
    F_pz   = wrench_ext(3);
    tau_px = wrench_ext(4);
    tau_py = wrench_ext(5);

    % --- Prepare arguments for auto-generated functions ---
    % Create separate parameter vectors for each plane, now including h_app
    % Note: I_Ux is for roll, I_Uy is for pitch.
    params_arg_roll = [p.m_U,  p.I_Uy, p.I_Ux, p.l_U, p.m_S, p.I_S, p.r_S, p.g, p.h_app, p.b_theta, p.b_phi];
    params_arg_pitch = [p.m_U, p.I_Uy, p.I_Ux, p.l_U, p.m_S, p.I_S, p.r_S, p.g,p.h_app, p.b_theta, p.b_phi];
    
    external_vars_x = [F_py, F_pz, tau_px]; % For Roll dynamics
    external_vars_y = [F_px, F_pz, tau_py]; % For Pitch dynamics

    % --- X-Z Plane (Roll) Dynamics ---
    states_arg_x = [theta_x, dot_theta_x, dot_phi_x];
    inputs_arg_x = [tau_x];
    ddot_theta_x = copy_autogen_ddot_theta_x(states_arg_x, inputs_arg_x, params_arg_roll, external_vars_x);
    ddot_phi_x   = copy_autogen_ddot_phi_x(states_arg_x, inputs_arg_x, params_arg_roll, external_vars_x);
    

    % --- Y-Z Plane (Pitch) Dynamics ---
    states_arg_y = [theta_y, dot_theta_y, dot_phi_y];
    inputs_arg_y = [tau_y];
    ddot_theta_y = copy_autogen_ddot_theta_y(states_arg_y, inputs_arg_y, params_arg_pitch, external_vars_y);
    ddot_phi_y   = copy_autogen_ddot_phi_y(states_arg_y, inputs_arg_y, params_arg_pitch, external_vars_y);
    
    % --- Transversal Plane Dynamics (Yaw) ---
    % external forces at the center of the top surface are assumed not to produce yaw torque.
    ddot_theta_z = (tau_z - p.fz * dot_theta_z) / p.Iz;
    
    % --- Assemble the state derivative vector dx ---
    dx = [
        dot_theta_x;    % dx(1) = d(theta_x)/dt
        dot_theta_y;    % dx(2) = d(theta_y)/dt
        dot_theta_z;    % dx(3) = d(theta_z)/dt
        dot_phi_x;      % dx(4) = d(phi_x)/dt
        dot_phi_y;      % dx(5) = d(phi_y)/dt
        ddot_theta_x;   % dx(6) = d(dot_theta_x)/dt
        ddot_theta_y;   % dx(7) = d(dot_theta_y)/dt
        ddot_theta_z;   % dx(8) = d(dot_theta_z)/dt
        ddot_phi_x;     % dx(9) = d(dot_phi_x)/dt
        ddot_phi_y;     % dx(10)= d(dot_phi_y)/dt
    ];
end
